simulink model "StandTurn_Balance_zhengqi"  (R2021a)
settings: Solver=FixedStepDiscrete  StartTime=0.0  StopTime=inf  FixedStep=0.0005  RelTol=1e-3
libraries: simulink x13, IFR_StackLiteDualDrive_SimulinkLib x4
settings Model: Creator=ysl  LastModifiedBy=ysl
settings OptimizationCC: DefaultParameterBehavior=Inlined  EnhancedBackFolding=on  PassReuseOutputArgsAs=Individual arguments  ZeroExternalMemoryAtStartup=off  ZeroInternalMemoryAtStartup=off  OptimizeBlockOrder=speed  DifferentSizesBufferReuse=on  OptimizationCustomize=off  EfficientTunableParamExpr=on
settings DebuggingCC: ParameterTunabilityLossMsg=error
settings SFSimCC: MATLABDynamicMemAlloc=off
settings RTWCC: Description=IFR StackLite-DualDrive Base on stm32f405RGT6  SystemTargetFile=stacklite_dualdrive.tlc  TemplateMakefile=stacklite_dualdrive.tmf  GenerateReport=on
settings CodeAppCC: ForceParamTrailComments=on  IgnoreCustomStorageClasses=off  OperatorAnnotations=on  SimulinkDataObjDesc=on  SFDataObjDesc=on  InsertBlockDesc=on
settings STFCustomTargetCC: TargetLangStandard=C99 (ISO)  MultiwordLength=256  ParMdlRefBuildCompliant=on  CompOptLevelCompliant=on  CombineOutputUpdateFcns=on  ERTCustomFileBanners=on  SupportContinuousTime=off  SupportNonInlinedSFcns=off  RemoveResetFunc=on  MATLABClassNameForMDSCustomization=Simulink.SoftwareTarget.ERTCustomization  CPPClassGenCompliant=on  GRTInterface=off  UseToolchainInfoCompliant=off  SystemTargetFile=stacklite_dualdrive.tlc
settings ERTTargetCC: TargetLangStandard=C99 (ISO)  ConcurrentExecutionCompliant=off  ModelStepFunctionPrototypeControlCompliant=off  UseToolchainInfoCompliant=off  InlinedParameterPlacement=NonHierarchical  ERTCustomFileTemplate=example_file_process.tlc

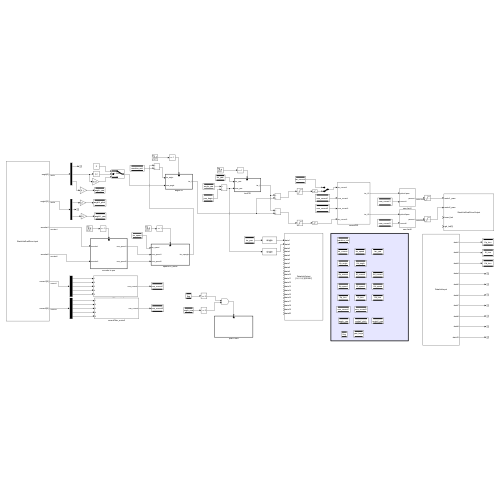
[thumbnail: Simulink's stored preview of the top-level diagram]
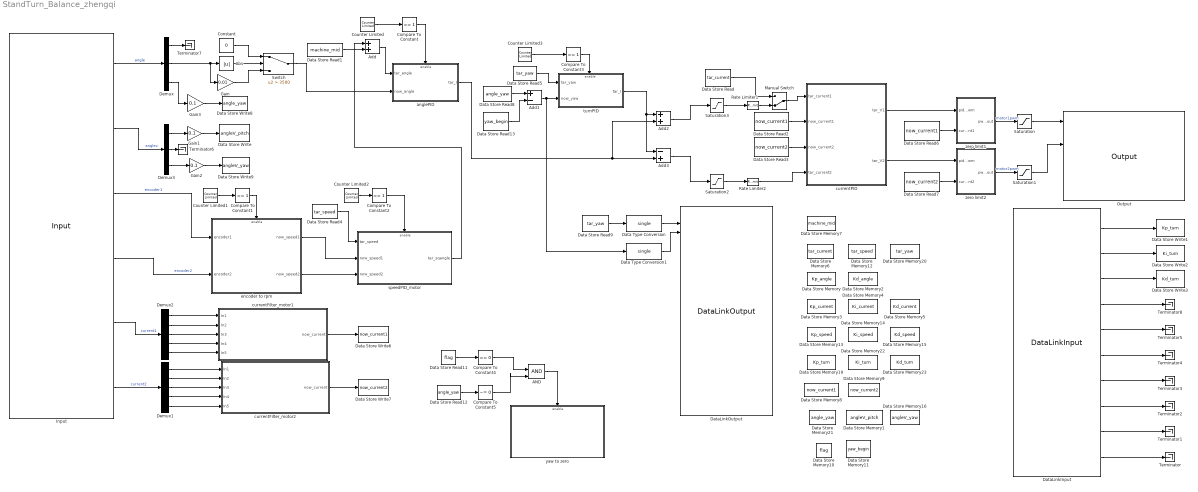
== system StandTurn_Balance_zhengqi ==
  AND : Logic  IconShape=distinctive  AllPortsSameDT=off  OutDataTypeStr=boolean
  Abs : Abs
  Add : Sum
  Add1 : Sum  Inputs=+-
  Add2 : Sum
  Add3 : Sum  Inputs=-+
  Compare To Constant{,1..3} (4 alike) : simulink/Logic and Bit Operations/Compare To Constant  relop===  const=1  OutDataTypeStr=boolean
  Compare To Constant4 : simulink/Logic and Bit Operations/Compare To Constant  relop===  const=0  OutDataTypeStr=boolean
  Compare To Constant5 : simulink/Logic and Bit Operations/Compare To Constant  relop=~=  const=0  OutDataTypeStr=boolean
  Constant : Constant  Value=0
  Counter Limited{,1..3} (4 alike) : simulink/Sources/Counter Limited  uplimit=1  tsamp=-1
  Data Store Memory : DataStoreMemory  DataStoreName=Kp_angle  ReadBeforeWriteMsg=warning  WriteAfterWriteMsg=warning  WriteAfterReadMsg=warning  ShowAdditionalParam=off
  Data Store Memory1 : DataStoreMemory  DataStoreName=angleV_pitch  ReadBeforeWriteMsg=warning  WriteAfterWriteMsg=warning  WriteAfterReadMsg=warning  ShowAdditionalParam=off
  Data Store Memory10 : DataStoreMemory  DataStoreName=flag  ReadBeforeWriteMsg=warning  WriteAfterWriteMsg=warning  WriteAfterReadMsg=warning  ShowAdditionalParam=off
  Data Store Memory11 : DataStoreMemory  DataStoreName=yaw_begin  ReadBeforeWriteMsg=warning  WriteAfterWriteMsg=warning  WriteAfterReadMsg=warning  ShowAdditionalParam=off
  Data Store Memory12 : DataStoreMemory  DataStoreName=tar_speed  ReadBeforeWriteMsg=warning  WriteAfterWriteMsg=warning  WriteAfterReadMsg=warning  ShowAdditionalParam=off
  Data Store Memory13 : DataStoreMemory  DataStoreName=Kp_speed  ReadBeforeWriteMsg=warning  WriteAfterWriteMsg=warning  WriteAfterReadMsg=warning  ShowAdditionalParam=off
  Data Store Memory14 : DataStoreMemory  DataStoreName=Ki_speed  ReadBeforeWriteMsg=warning  WriteAfterWriteMsg=warning  WriteAfterReadMsg=warning  ShowAdditionalParam=off
  Data Store Memory15 : DataStoreMemory  DataStoreName=Kd_speed  ReadBeforeWriteMsg=warning  WriteAfterWriteMsg=warning  WriteAfterReadMsg=warning  ShowAdditionalParam=off
  Data Store Memory16 : DataStoreMemory  DataStoreName=angleV_yaw  ReadBeforeWriteMsg=warning  WriteAfterWriteMsg=warning  WriteAfterReadMsg=warning  ShowAdditionalParam=off
  Data Store Memory19 : DataStoreMemory  DataStoreName=Kp_turn  ReadBeforeWriteMsg=warning  WriteAfterWriteMsg=warning  WriteAfterReadMsg=warning  ShowAdditionalParam=off
  Data Store Memory2 : DataStoreMemory  DataStoreName=Kd_angle  ReadBeforeWriteMsg=warning  WriteAfterWriteMsg=warning  WriteAfterReadMsg=warning  ShowAdditionalParam=off
  Data Store Memory20 : DataStoreMemory  DataStoreName=tar_yaw  ReadBeforeWriteMsg=warning  WriteAfterWriteMsg=warning  WriteAfterReadMsg=warning  ShowAdditionalParam=off
  Data Store Memory21 : DataStoreMemory  DataStoreName=angle_yaw  ReadBeforeWriteMsg=warning  WriteAfterWriteMsg=warning  WriteAfterReadMsg=warning  ShowAdditionalParam=off
  Data Store Memory22 : DataStoreMemory  DataStoreName=Ki_turn  ReadBeforeWriteMsg=warning  WriteAfterWriteMsg=warning  WriteAfterReadMsg=warning  ShowAdditionalParam=off
  Data Store Memory23 : DataStoreMemory  DataStoreName=Kd_turn  ReadBeforeWriteMsg=warning  WriteAfterWriteMsg=warning  WriteAfterReadMsg=warning  ShowAdditionalParam=off
  Data Store Memory3 : DataStoreMemory  DataStoreName=Kp_current  ReadBeforeWriteMsg=warning  WriteAfterWriteMsg=warning  WriteAfterReadMsg=warning  ShowAdditionalParam=off
  Data Store Memory4 : DataStoreMemory  DataStoreName=Ki_current  ReadBeforeWriteMsg=warning  WriteAfterWriteMsg=warning  WriteAfterReadMsg=warning  ShowAdditionalParam=off
  Data Store Memory5 : DataStoreMemory  DataStoreName=Kd_current  ReadBeforeWriteMsg=warning  WriteAfterWriteMsg=warning  WriteAfterReadMsg=warning  ShowAdditionalParam=off
  Data Store Memory6 : DataStoreMemory  DataStoreName=tar_current  ReadBeforeWriteMsg=warning  WriteAfterWriteMsg=warning  WriteAfterReadMsg=warning  ShowAdditionalParam=off
  Data Store Memory7 : DataStoreMemory  DataStoreName=machine_mid  ReadBeforeWriteMsg=warning  WriteAfterWriteMsg=warning  WriteAfterReadMsg=warning  ShowAdditionalParam=off
  Data Store Memory8 : DataStoreMemory  DataStoreName=now_current1  ReadBeforeWriteMsg=warning  WriteAfterWriteMsg=warning  WriteAfterReadMsg=warning  ShowAdditionalParam=off
  Data Store Memory9 : DataStoreMemory  DataStoreName=now_current2  ReadBeforeWriteMsg=warning  WriteAfterWriteMsg=warning  WriteAfterReadMsg=warning  ShowAdditionalParam=off
  Data Store Read : DataStoreRead  DataStoreName=tar_current  IndexOptions=Index vector (dialog)  Indices=1  OutputSizes=1
  Data Store Read1 : DataStoreRead  DataStoreName=machine_mid  IndexOptions=Index vector (dialog)  Indices=1  OutputSizes=1
  Data Store Read11 : DataStoreRead  DataStoreName=flag  IndexOptions=Index vector (dialog)  Indices=1  OutputSizes=1
  Data Store Read12 : DataStoreRead  DataStoreName=angle_yaw  IndexOptions=Index vector (dialog)  Indices=1  OutputSizes=1
  Data Store Read13 : DataStoreRead  DataStoreName=yaw_begin  IndexOptions=Index vector (dialog)  Indices=1  OutputSizes=1
  Data Store Read2 : DataStoreRead  DataStoreName=now_current1  IndexOptions=Index vector (dialog)  Indices=1  OutputSizes=1
  Data Store Read3 : DataStoreRead  DataStoreName=now_current2  IndexOptions=Index vector (dialog)  Indices=1  OutputSizes=1
  Data Store Read4 : DataStoreRead  DataStoreName=tar_speed  IndexOptions=Index vector (dialog)  Indices=1  OutputSizes=1
  Data Store Read5 : DataStoreRead  DataStoreName=tar_yaw  IndexOptions=Index vector (dialog)  Indices=1  OutputSizes=1
  Data Store Read6 : DataStoreRead  DataStoreName=now_current1  IndexOptions=Index vector (dialog)  Indices=1  OutputSizes=1
  Data Store Read7 : DataStoreRead  DataStoreName=now_current2  IndexOptions=Index vector (dialog)  Indices=1  OutputSizes=1
  Data Store Read8 : DataStoreRead  DataStoreName=angle_yaw  IndexOptions=Index vector (dialog)  Indices=1  OutputSizes=1
  Data Store Read9 : DataStoreRead  DataStoreName=tar_yaw  IndexOptions=Index vector (dialog)  Indices=1  OutputSizes=1
  Data Store Write : DataStoreWrite  DataStoreName=angleV_pitch  IndexOptions=Index vector (dialog)  Indices=1  OutputSizes=1
  Data Store Write1 : DataStoreWrite  DataStoreName=Kp_turn  IndexOptions=Index vector (dialog)  Indices=1  OutputSizes=1
  Data Store Write2 : DataStoreWrite  DataStoreName=Ki_turn  IndexOptions=Index vector (dialog)  Indices=1  OutputSizes=1
  Data Store Write3 : DataStoreWrite  DataStoreName=Kd_turn  IndexOptions=Index vector (dialog)  Indices=1  OutputSizes=1
  Data Store Write6 : DataStoreWrite  DataStoreName=now_current1  IndexOptions=Index vector (dialog)  Indices=1  OutputSizes=1
  Data Store Write7 : DataStoreWrite  DataStoreName=now_current2  IndexOptions=Index vector (dialog)  Indices=1  OutputSizes=1
  Data Store Write8 : DataStoreWrite  DataStoreName=angle_yaw  IndexOptions=Index vector (dialog)  Indices=1  OutputSizes=1
  Data Store Write9 : DataStoreWrite  DataStoreName=angleV_yaw  IndexOptions=Index vector (dialog)  Indices=1  OutputSizes=1
  Data Type Conversion : DataTypeConversion  OutDataTypeStr=single
  Data Type Conversion1 : DataTypeConversion  OutDataTypeStr=single
  DataLinkInput : IFR_StackLiteDualDrive_SimulinkLib/DataLinkInput
      settings: SourceProductName=IFR_StackLiteDualDrive_SimulinkLib_V1.0
  DataLinkOutput : IFR_StackLiteDualDrive_SimulinkLib/DataLinkOutput  id='BalanceUnname'  key='IFR00'
      settings: SourceProductName=IFR_StackLiteDualDrive_SimulinkLib_V1.0
  Demux : Demux  Outputs=3
  Demux1 : Demux  Outputs=5
  Demux2 : Demux  Outputs=5
  Demux3 : Demux  Outputs=3
  Gain : Gain  Gain=0.01
  Gain1 : Gain  Gain=0.1
  Gain2 : Gain  Gain=0.1
  Gain3 : Gain  Gain=0.1
  Input : IFR_StackLiteDualDrive_SimulinkLib/Input  Priority=0
      settings: SourceProductName=IFR_StackLiteDualDrive_SimulinkLib_V1.0
  Manual Switch : ManualSwitch  CurrentSetting=0
  Output : IFR_StackLiteDualDrive_SimulinkLib/Output  Priority=255
      settings: SourceProductName=IFR_StackLiteDualDrive_SimulinkLib_V1.0
  Rate Limiter1 : RateLimiter  RisingSlewLimit=10000  FallingSlewLimit=-10000  SampleTimeMode=inherited
  Rate Limiter2 : RateLimiter  RisingSlewLimit=10000  FallingSlewLimit=-10000  SampleTimeMode=inherited
  Saturation : Saturate  UpperLimit=4200  LowerLimit=-4200
  Saturation1 : Saturate  UpperLimit=4200  LowerLimit=-4200
  Saturation2 : Saturate  UpperLimit=2048  LowerLimit=-2048  OutDataTypeStr=int16
  Saturation3 : Saturate  UpperLimit=2048  LowerLimit=-2048  OutDataTypeStr=int16
  Switch : Switch  Criteria=u2 > Threshold  Threshold=3500
  Terminator{,1..8} (9 alike) : Terminator
  anglePID : Subsystem
  currentFilter_motor1 : Subsystem
  currentFilter_motor2 : Subsystem
  currentPID : Subsystem
  encoder to rpm : Subsystem
  speedPID_motor : Subsystem
  turnPID : Subsystem
  yaw to zero : Subsystem
  zero limit1 : Subsystem
  zero limit2 : Subsystem
  wires:
  Input/5 -> Demux2/1  "current1"
  Saturation1/1 -> Output/2
  Saturation2/1 -> Rate Limiter2/1
  Data Store Read3/1 -> currentPID/3(now_current2)
  Rate Limiter2/1 -> currentPID/4(tar_current2)
  Input/1 -> Demux/1  "angle"
  currentFilter_motor2/1(now_current) -> Data Store Write7/1
  Manual Switch/1 -> currentPID/1(tar_current1)
  Compare To Constant1/1 -> encoder to rpm/Enable
  Demux1/4 -> currentFilter_motor2/4(In4)
  Counter Limited1/1 -> Compare To Constant1/1
  Demux2/2 -> currentFilter_motor1/2(In2)
  zero limit2/1(pwmout) -> Saturation1/1  "motor2pwm"
  Demux1/1 -> currentFilter_motor2/1(In1)
  Demux2/5 -> currentFilter_motor1/5(In5)
  Input/3 -> encoder to rpm/1(encoder1)  "encoder1"
  Saturation3/1 -> Rate Limiter1/1
  Saturation/1 -> Output/1
  Demux1/3 -> currentFilter_motor2/3(In3)
  Input/6 -> Demux1/1  "current2"
  Demux2/3 -> currentFilter_motor1/3(In3)
  Demux/3 -> Gain3/1
  currentPID/2(tar_V2) -> zero limit2/1(pidout2pwm)
  Input/2 -> Demux3/1  "anglev"
  Demux3/2 -> Terminator6/1
  Demux2/1 -> currentFilter_motor1/1(In1)
  Demux1/5 -> currentFilter_motor2/5(In5)
  Input/4 -> encoder to rpm/2(encoder2)  "encoder2"
  currentPID/1(tar_V1) -> zero limit1/1(pidout1pwm)
  Demux1/2 -> currentFilter_motor2/2(In2)
  Data Store Read2/1 -> currentPID/2(now_current1)
  Data Store Read7/1 -> zero limit2/2(current2)
  currentFilter_motor1/1(now_current) -> Data Store Write6/1
  Rate Limiter1/1 -> Manual Switch/2
  Demux2/4 -> currentFilter_motor1/4(In4)
  zero limit1/1(pwmout) -> Saturation/1  "motor1pwm"
  Data Store Read/1 -> Manual Switch/1
  Data Store Read6/1 -> zero limit1/2(current1)
  Add/1 -> anglePID/1(tar_angle)
  Abs/1 -> Switch/2
  Gain/1 -> Switch/3
  Constant/1 -> Switch/1
  Demux/2 -> Gain/1, Abs/1
  Counter Limited/1 -> Compare To Constant/1
  Switch/1 -> anglePID/2(now_angle)
  Data Store Read1/1 -> Add/2
  Compare To Constant/1 -> anglePID/Enable
  Demux/1 -> Terminator7/1
  speedPID_motor/1(tar_sqangle) -> Add/1
  Demux3/1 -> Gain1/1
  Gain1/1 -> Data Store Write/1
  Data Store Read4/1 -> speedPID_motor/1(tar_speed)
  Counter Limited2/1 -> Compare To Constant2/1
  Compare To Constant2/1 -> speedPID_motor/Enable
  encoder to rpm/1(now_speed1) -> speedPID_motor/2(now_speed1)
  encoder to rpm/2(now_speed2) -> speedPID_motor/3(now_speed2)
  Data Store Read5/1 -> turnPID/1(tar_yaw)
  Demux3/3 -> Gain2/1
  Gain2/1 -> Data Store Write9/1
  Gain3/1 -> Data Store Write8/1
  turnPID/1(tar_I) -> Add3/1, Add2/1
  anglePID/1(tar_I) -> Add2/2, Add3/2
  Add2/1 -> Saturation3/1
  Add3/1 -> Saturation2/1
  Compare To Constant3/1 -> turnPID/Enable
  Counter Limited3/1 -> Compare To Constant3/1
  Data Store Read9/1 -> Data Type Conversion/1
  Data Type Conversion/1 -> DataLinkOutput/1
  Add1/1 -> Data Type Conversion1/1, turnPID/2(now_yaw)
  Data Type Conversion1/1 -> DataLinkOutput/2
  Data Store Read11/1 -> Compare To Constant4/1
  Data Store Read12/1 -> Compare To Constant5/1
  Compare To Constant4/1 -> AND/1
  Compare To Constant5/1 -> AND/2
  AND/1 -> yaw to zero/Enable
  Data Store Read8/1 -> Add1/1
  Data Store Read13/1 -> Add1/2
  DataLinkInput/10 -> Terminator/1
  DataLinkInput/9 -> Terminator1/1
  DataLinkInput/8 -> Terminator2/1
  DataLinkInput/7 -> Terminator3/1
  DataLinkInput/6 -> Terminator4/1
  DataLinkInput/5 -> Terminator5/1
  DataLinkInput/4 -> Terminator8/1
  DataLinkInput/1 -> Data Store Write1/1
  DataLinkInput/2 -> Data Store Write2/1
  DataLinkInput/3 -> Data Store Write3/1

== system StandTurn_Balance_zhengqi/anglePID ==
  tar_angle : Inport
  now_angle : Inport  Port=2
  Enable : EnablePort
  Add : Sum  OutDataTypeStr=double
  Add1 : Sum  Inputs=+-
  D : Subsystem
  P : Subsystem
  tar_I : Outport
  wires:
  Add/1 -> tar_I/1
  D/1(Out1) -> Add/2
  now_angle/1 -> Add1/2
  tar_angle/1 -> Add1/1
  P/1(Out1) -> Add/1
  Add1/1 -> P/1(error)

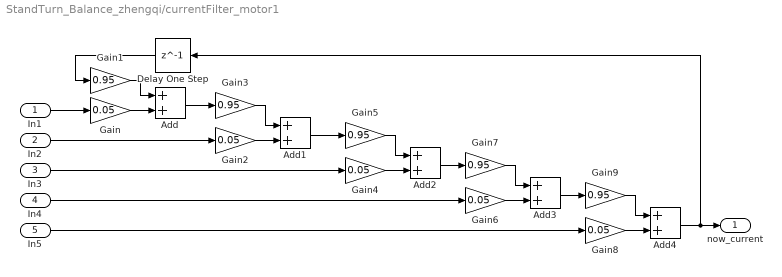
== system StandTurn_Balance_zhengqi/currentFilter_motor1 ==
  In1 : Inport
  In2 : Inport  Port=2
  In3 : Inport  Port=3
  In4 : Inport  Port=4
  In5 : Inport  Port=5
  Add{,1..4} (5 alike) : Sum
  Delay One Step : Delay  DelayLength=1
  Gain{,2,4,6,8} (5 alike) : Gain  Gain=0.05  OutDataTypeStr=single
  Gain{1,3,5,7,9} (5 alike) : Gain  Gain=0.95  OutDataTypeStr=single
  now_current : Outport
  wires:
  Gain1/1 -> Add/1
  Gain5/1 -> Add2/1
  Gain/1 -> Add/2
  Gain3/1 -> Add1/1
  In2/1 -> Gain2/1
  Gain2/1 -> Add1/2
  Delay One Step/1 -> Gain1/1
  In1/1 -> Gain/1
  Add/1 -> Gain3/1
  Gain4/1 -> Add2/2
  In4/1 -> Gain6/1
  Add1/1 -> Gain5/1
  Gain9/1 -> Add4/1
  Add2/1 -> Gain7/1
  Gain8/1 -> Add4/2
  Gain7/1 -> Add3/1
  Add4/1 -> now_current/1, Delay One Step/1
  Gain6/1 -> Add3/2
  Add3/1 -> Gain9/1
  In5/1 -> Gain8/1
  In3/1 -> Gain4/1

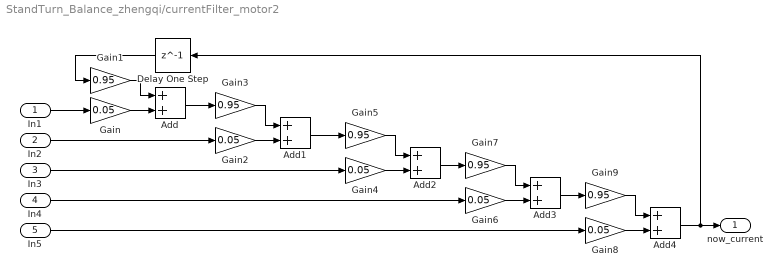
== system StandTurn_Balance_zhengqi/currentFilter_motor2 ==
  In1 : Inport
  In2 : Inport  Port=2
  In3 : Inport  Port=3
  In4 : Inport  Port=4
  In5 : Inport  Port=5
  Add{,1..4} (5 alike) : Sum
  Delay One Step : Delay  DelayLength=1
  Gain{,2,4,6,8} (5 alike) : Gain  Gain=0.05  OutDataTypeStr=single
  Gain{1,3,5,7,9} (5 alike) : Gain  Gain=0.95  OutDataTypeStr=single
  now_current : Outport
  wires:
  In3/1 -> Gain4/1
  In5/1 -> Gain8/1
  Add3/1 -> Gain9/1
  Gain6/1 -> Add3/2
  Add4/1 -> Delay One Step/1, now_current/1
  Gain7/1 -> Add3/1
  Gain8/1 -> Add4/2
  Add2/1 -> Gain7/1
  Gain9/1 -> Add4/1
  Add1/1 -> Gain5/1
  In4/1 -> Gain6/1
  Gain4/1 -> Add2/2
  Add/1 -> Gain3/1
  In1/1 -> Gain/1
  Delay One Step/1 -> Gain1/1
  Gain2/1 -> Add1/2
  In2/1 -> Gain2/1
  Gain3/1 -> Add1/1
  Gain/1 -> Add/2
  Gain5/1 -> Add2/1
  Gain1/1 -> Add/1

== system StandTurn_Balance_zhengqi/currentPID ==
  tar_current1 : Inport
  now_current1 : Inport  Port=2
  now_current2 : Inport  Port=3
  tar_current2 : Inport  Port=4
  currentPID_motor1 : Subsystem
  currentPID_motor2 : Subsystem
  tar_V1 : Outport
  tar_V2 : Outport  Port=2
  wires:
  tar_current1/1 -> currentPID_motor1/1(tar_current)
  now_current1/1 -> currentPID_motor1/2(now_current)
  currentPID_motor1/1(tar_V) -> tar_V1/1
  now_current2/1 -> currentPID_motor2/2(now_current)
  currentPID_motor2/1(tar_V) -> tar_V2/1
  tar_current2/1 -> currentPID_motor2/1(tar_current)

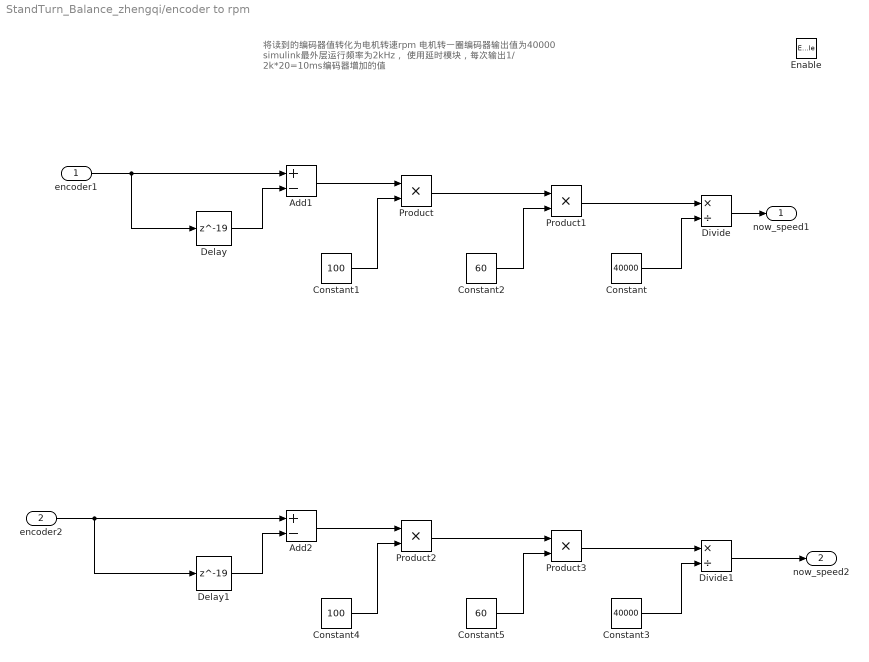
== system StandTurn_Balance_zhengqi/encoder to rpm ==
  note: 将读到的编码器值转化为电机转速rpm
      | 电机转一圈编码器输出值为40000
      | simulink最外层运行频率为2kHz，
      | 使用延时模块，每次输出1/ 2k*20=10ms编码器增加的值
  encoder1 : Inport
  encoder2 : Inport  Port=2
  Enable : EnablePort
  Add1 : Sum  Inputs=+-
  Add2 : Sum  Inputs=+-
  Constant : Constant  Value=40000  OutDataTypeStr=single
  Constant1 : Constant  Value=100  OutDataTypeStr=single
  Constant2 : Constant  Value=60  OutDataTypeStr=single
  Constant3 : Constant  Value=40000  OutDataTypeStr=single
  Constant4 : Constant  Value=100  OutDataTypeStr=single
  Constant5 : Constant  Value=60  OutDataTypeStr=single
  Delay : Delay  DelayLength=19
  Delay1 : Delay  DelayLength=19
  Divide : Product  Inputs=*/  OutDataTypeStr=single
  Divide1 : Product  Inputs=*/  OutDataTypeStr=single
  Product{,1..3} (4 alike) : Product  OutDataTypeStr=single
  now_speed1 : Outport
  now_speed2 : Outport  Port=2
  wires:
  Product1/1 -> Divide/1
  Product/1 -> Product1/1
  Constant/1 -> Divide/2
  encoder1/1 -> Add1/1, Delay/1
  Add2/1 -> Product2/1
  Delay1/1 -> Add2/2
  encoder2/1 -> Add2/1, Delay1/1
  Constant1/1 -> Product/2
  Add1/1 -> Product/1
  Constant2/1 -> Product1/2
  Delay/1 -> Add1/2
  Divide1/1 -> now_speed2/1
  Product2/1 -> Product3/1
  Constant4/1 -> Product2/2
  Product3/1 -> Divide1/1
  Constant5/1 -> Product3/2
  Divide/1 -> now_speed1/1
  Constant3/1 -> Divide1/2

== system StandTurn_Balance_zhengqi/speedPID_motor ==
  tar_speed : Inport
  now_speed1 : Inport  Port=2
  now_speed2 : Inport  Port=3
  Enable : EnablePort
  Subsystem2 : Subsystem
  tar_sqangle : Outport
  wires:
  Subsystem2/1(tar_sqangle) -> tar_sqangle/1
  now_speed2/1 -> Subsystem2/3(now_speed2)
  now_speed1/1 -> Subsystem2/2(now_speed1)
  tar_speed/1 -> Subsystem2/1(tar_speed)

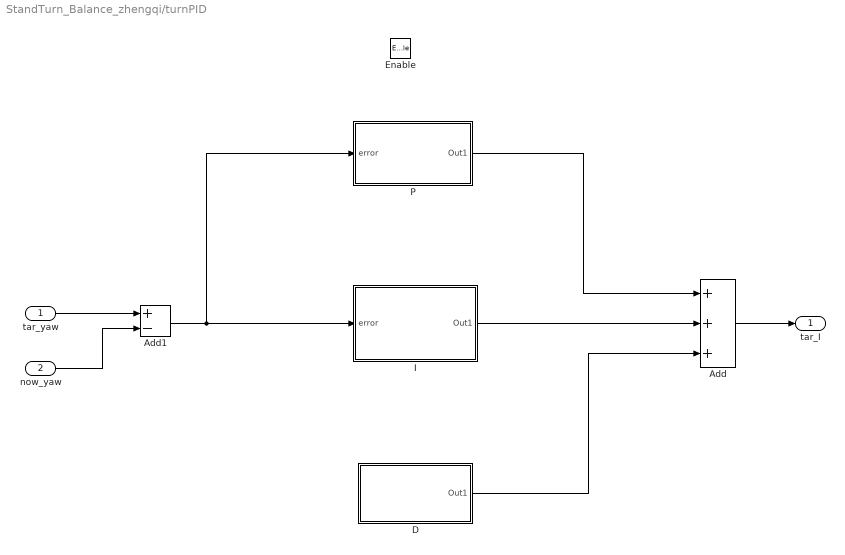
== system StandTurn_Balance_zhengqi/turnPID ==
  tar_yaw : Inport
  now_yaw : Inport  Port=2
  Enable : EnablePort
  Add : Sum  Inputs=+++  OutDataTypeStr=double
  Add1 : Sum  Inputs=+-
  D : Subsystem
  I : Subsystem
  P : Subsystem
  tar_I : Outport
  wires:
  I/1(Out1) -> Add/2
  tar_yaw/1 -> Add1/1
  now_yaw/1 -> Add1/2
  P/1(Out1) -> Add/1
  Add1/1 -> I/1(error), P/1(error)
  Add/1 -> tar_I/1
  D/1(Out1) -> Add/3

== system StandTurn_Balance_zhengqi/yaw to zero ==
  Enable : EnablePort
  Constant : Constant
  Data Store Read : DataStoreRead  DataStoreName=angle_yaw  IndexOptions=Index vector (dialog)  Indices=1  OutputSizes=1
  Data Store Write : DataStoreWrite  DataStoreName=yaw_begin  IndexOptions=Index vector (dialog)  Indices=1  OutputSizes=1
  Data Store Write1 : DataStoreWrite  DataStoreName=flag  IndexOptions=Index vector (dialog)  Indices=1  OutputSizes=1
  wires:
  Data Store Read/1 -> Data Store Write/1
  Constant/1 -> Data Store Write1/1

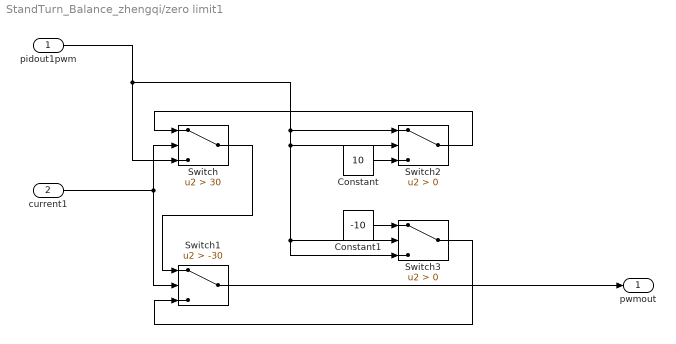
== system StandTurn_Balance_zhengqi/zero limit1 ==
  pidout1pwm : Inport
  current1 : Inport  Port=2
  Constant : Constant  Value=10  OutDataTypeStr=int16
  Constant1 : Constant  Value=-10  OutDataTypeStr=int16
  Switch : Switch  Criteria=u2 > Threshold  Threshold=30  OutDataTypeStr=int16
  Switch1 : Switch  Criteria=u2 > Threshold  Threshold=-30  OutDataTypeStr=int16
  Switch2 : Switch  Criteria=u2 > Threshold  OutDataTypeStr=int16
  Switch3 : Switch  Criteria=u2 > Threshold  OutDataTypeStr=int16
  pwmout : Outport
  wires:
  Switch1/1 -> pwmout/1
  Switch2/1 -> Switch/1
  Switch3/1 -> Switch1/3
  Switch/1 -> Switch1/1
  Constant/1 -> Switch2/3
  pidout1pwm/1 -> Switch2/2, Switch3/2, Switch3/3, Switch2/1, Switch/3
  current1/1 -> Switch1/2, Switch/2
  Constant1/1 -> Switch3/1

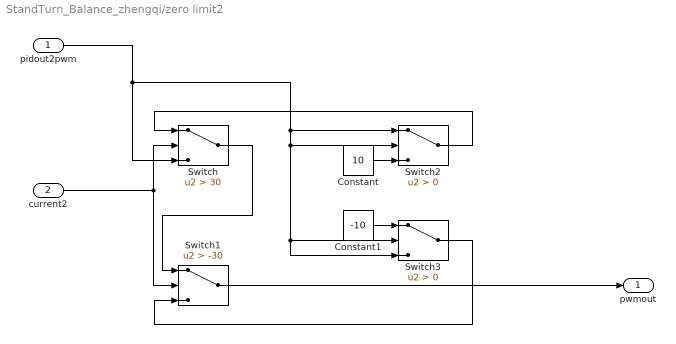
== system StandTurn_Balance_zhengqi/zero limit2 ==
  pidout2pwm : Inport
  current2 : Inport  Port=2
  Constant : Constant  Value=10  OutDataTypeStr=int16
  Constant1 : Constant  Value=-10  OutDataTypeStr=int16
  Switch : Switch  Criteria=u2 > Threshold  Threshold=30  OutDataTypeStr=int16
  Switch1 : Switch  Criteria=u2 > Threshold  Threshold=-30  OutDataTypeStr=int16
  Switch2 : Switch  Criteria=u2 > Threshold  OutDataTypeStr=int16
  Switch3 : Switch  Criteria=u2 > Threshold  OutDataTypeStr=int16
  pwmout : Outport
  wires:
  Constant1/1 -> Switch3/1
  current2/1 -> Switch/2, Switch1/2
  pidout2pwm/1 -> Switch/3, Switch2/1, Switch3/3, Switch3/2, Switch2/2
  Constant/1 -> Switch2/3
  Switch/1 -> Switch1/1
  Switch3/1 -> Switch1/3
  Switch2/1 -> Switch/1
  Switch1/1 -> pwmout/1

== system StandTurn_Balance_zhengqi/anglePID/D ==
  Constant2 : Constant  Value=0.1
  Data Store Read : DataStoreRead  DataStoreName=angleV_pitch  IndexOptions=Index vector (dialog)  Indices=1  OutputSizes=1
  Data Store Read2 : DataStoreRead  DataStoreName=Kd_angle  IndexOptions=Index vector (dialog)  Indices=1  OutputSizes=1
  Manual Switch2 : ManualSwitch
  Product2 : Product
  Out1 : Outport
  wires:
  Data Store Read/1 -> Product2/2
  Product2/1 -> Out1/1
  Data Store Read2/1 -> Manual Switch2/2
  Manual Switch2/1 -> Product2/1
  Constant2/1 -> Manual Switch2/1

== system StandTurn_Balance_zhengqi/anglePID/P ==
  error : Inport
  Constant : Constant  Value=70
  Data Store Read : DataStoreRead  DataStoreName=Kp_angle  IndexOptions=Index vector (dialog)  Indices=1  OutputSizes=1
  Manual Switch : ManualSwitch
  Product : Product
  Out1 : Outport
  wires:
  error/1 -> Product/2
  Manual Switch/1 -> Product/1
  Data Store Read/1 -> Manual Switch/2
  Constant/1 -> Manual Switch/1
  Product/1 -> Out1/1

== system StandTurn_Balance_zhengqi/currentPID/currentPID_motor1 ==
  tar_current : Inport
  now_current : Inport  Port=2
  Add : Sum  Inputs=+++  OutDataTypeStr=double
  Add1 : Sum  Inputs=+-
  D : Subsystem
  I : Subsystem
  P : Subsystem
  tar_V : Outport
  wires:
  I/1(Out1) -> Add/2
  tar_current/1 -> Add1/1
  now_current/1 -> Add1/2
  P/1(Out1) -> Add/1
  Add1/1 -> D/1(error), I/1(error), P/1(error)
  D/1(Out1) -> Add/3
  Add/1 -> tar_V/1

== system StandTurn_Balance_zhengqi/currentPID/currentPID_motor2 ==
  tar_current : Inport
  now_current : Inport  Port=2
  Add : Sum  Inputs=+++  OutDataTypeStr=double
  Add1 : Sum  Inputs=+-
  D : Subsystem
  I : Subsystem
  P : Subsystem
  tar_V : Outport
  wires:
  Add/1 -> tar_V/1
  D/1(Out1) -> Add/3
  Add1/1 -> P/1(error), I/1(error), D/1(error)
  P/1(Out1) -> Add/1
  now_current/1 -> Add1/2
  tar_current/1 -> Add1/1
  I/1(Out1) -> Add/2

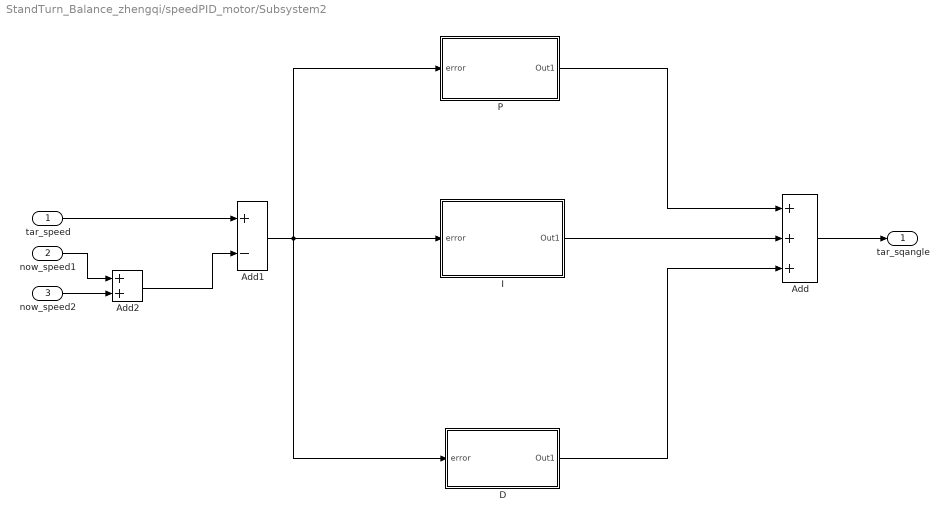
== system StandTurn_Balance_zhengqi/speedPID_motor/Subsystem2 ==
  tar_speed : Inport
  now_speed1 : Inport  Port=2
  now_speed2 : Inport  Port=3
  Add : Sum  Inputs=+++  OutDataTypeStr=double
  Add1 : Sum  Inputs=+-
  Add2 : Sum
  D : Subsystem
  I : Subsystem
  P : Subsystem
  tar_sqangle : Outport
  wires:
  Add2/1 -> Add1/2
  now_speed2/1 -> Add2/2
  now_speed1/1 -> Add2/1
  I/1(Out1) -> Add/2
  Add1/1 -> I/1(error), D/1(error), P/1(error)
  P/1(Out1) -> Add/1
  D/1(Out1) -> Add/3
  Add/1 -> tar_sqangle/1
  tar_speed/1 -> Add1/1

== system StandTurn_Balance_zhengqi/turnPID/D ==
  Constant2 : Constant  Value=0.1
  Data Store Read : DataStoreRead  DataStoreName=angleV_yaw  IndexOptions=Index vector (dialog)  Indices=1  OutputSizes=1
  Data Store Read2 : DataStoreRead  DataStoreName=Kd_turn  IndexOptions=Index vector (dialog)  Indices=1  OutputSizes=1
  Manual Switch2 : ManualSwitch  CurrentSetting=0
  Product2 : Product
  Out1 : Outport
  wires:
  Data Store Read/1 -> Product2/2
  Product2/1 -> Out1/1
  Data Store Read2/1 -> Manual Switch2/2
  Manual Switch2/1 -> Product2/1
  Constant2/1 -> Manual Switch2/1

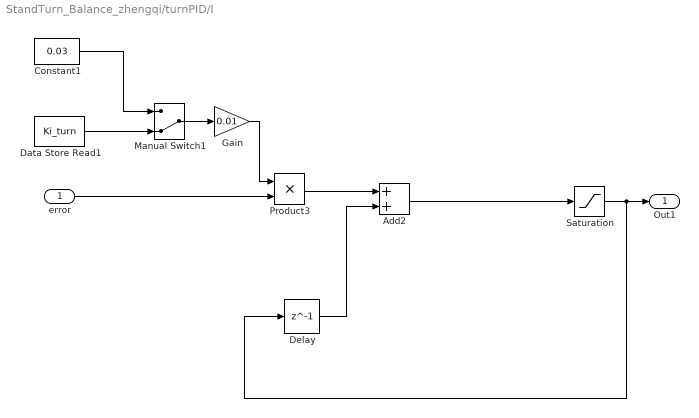
== system StandTurn_Balance_zhengqi/turnPID/I ==
  error : Inport
  Add2 : Sum
  Constant1 : Constant  Value=0.03
  Data Store Read1 : DataStoreRead  DataStoreName=Ki_turn  IndexOptions=Index vector (dialog)  Indices=1  OutputSizes=1
  Delay : Delay  DelayLength=1
  Gain : Gain  Gain=0.01
  Manual Switch1 : ManualSwitch  CurrentSetting=0
  Product3 : Product  OutDataTypeStr=single
  Saturation : Saturate  UpperLimit=2000  LowerLimit=-2000
  Out1 : Outport
  wires:
  Delay/1 -> Add2/2
  Gain/1 -> Product3/1
  Constant1/1 -> Manual Switch1/1
  Manual Switch1/1 -> Gain/1
  Data Store Read1/1 -> Manual Switch1/2
  Product3/1 -> Add2/1
  error/1 -> Product3/2
  Add2/1 -> Saturation/1
  Saturation/1 -> Delay/1, Out1/1

== system StandTurn_Balance_zhengqi/turnPID/P ==
  error : Inport
  Constant : Constant  Value=-30
  Data Store Read : DataStoreRead  DataStoreName=Kp_turn  IndexOptions=Index vector (dialog)  Indices=1  OutputSizes=1
  Manual Switch : ManualSwitch  CurrentSetting=0
  Product : Product
  Out1 : Outport
  wires:
  error/1 -> Product/2
  Manual Switch/1 -> Product/1
  Data Store Read/1 -> Manual Switch/2
  Constant/1 -> Manual Switch/1
  Product/1 -> Out1/1

== system StandTurn_Balance_zhengqi/currentPID/currentPID_motor1/D ==
  error : Inport
  Constant2 : Constant  Value=5
  Data Store Read2 : DataStoreRead  DataStoreName=Kd_current  IndexOptions=Index vector (dialog)  Indices=1  OutputSizes=1
  Difference : simulink/Discrete/Difference  ICPrevInput=0.0  OutMin=[]  OutMax=[]  OutDataType=fixdt(1, 16)  OutScaling=2^-10  DoSatur=off
  Manual Switch2 : ManualSwitch
  Product2 : Product
  Out1 : Outport
  wires:
  Difference/1 -> Product2/2
  Product2/1 -> Out1/1
  Data Store Read2/1 -> Manual Switch2/2
  Manual Switch2/1 -> Product2/1
  Constant2/1 -> Manual Switch2/1
  error/1 -> Difference/1

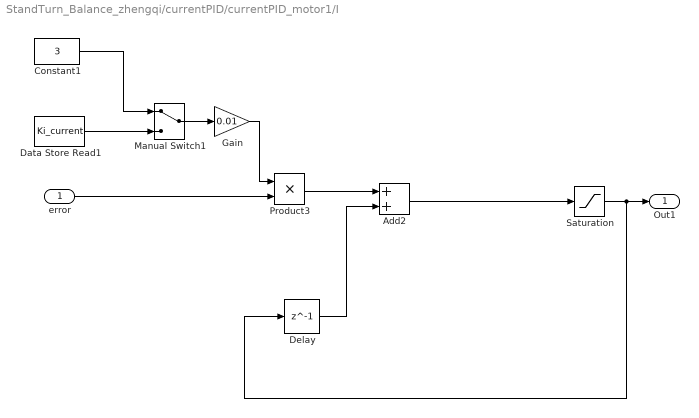
== system StandTurn_Balance_zhengqi/currentPID/currentPID_motor1/I ==
  error : Inport
  Add2 : Sum
  Constant1 : Constant  Value=3
  Data Store Read1 : DataStoreRead  DataStoreName=Ki_current  IndexOptions=Index vector (dialog)  Indices=1  OutputSizes=1
  Delay : Delay  DelayLength=1
  Gain : Gain  Gain=0.01
  Manual Switch1 : ManualSwitch
  Product3 : Product  OutDataTypeStr=single
  Saturation : Saturate  UpperLimit=2000  LowerLimit=-2000
  Out1 : Outport
  wires:
  Delay/1 -> Add2/2
  Gain/1 -> Product3/1
  Constant1/1 -> Manual Switch1/1
  Manual Switch1/1 -> Gain/1
  Data Store Read1/1 -> Manual Switch1/2
  Product3/1 -> Add2/1
  error/1 -> Product3/2
  Add2/1 -> Saturation/1
  Saturation/1 -> Delay/1, Out1/1

== system StandTurn_Balance_zhengqi/currentPID/currentPID_motor1/P ==
  error : Inport
  Constant : Constant  Value=7
  Data Store Read : DataStoreRead  DataStoreName=Kp_current  IndexOptions=Index vector (dialog)  Indices=1  OutputSizes=1
  Manual Switch : ManualSwitch
  Product : Product
  Out1 : Outport
  wires:
  error/1 -> Product/2
  Manual Switch/1 -> Product/1
  Data Store Read/1 -> Manual Switch/2
  Constant/1 -> Manual Switch/1
  Product/1 -> Out1/1

== system StandTurn_Balance_zhengqi/currentPID/currentPID_motor2/D ==
  error : Inport
  Constant2 : Constant  Value=4
  Data Store Read2 : DataStoreRead  DataStoreName=Kd_current  IndexOptions=Index vector (dialog)  Indices=1  OutputSizes=1
  Difference : simulink/Discrete/Difference  ICPrevInput=0.0  OutMin=[]  OutMax=[]  OutDataType=fixdt(1, 16)  OutScaling=2^-10  DoSatur=off
  Manual Switch2 : ManualSwitch
  Product2 : Product
  Out1 : Outport
  wires:
  error/1 -> Difference/1
  Constant2/1 -> Manual Switch2/1
  Manual Switch2/1 -> Product2/1
  Data Store Read2/1 -> Manual Switch2/2
  Product2/1 -> Out1/1
  Difference/1 -> Product2/2

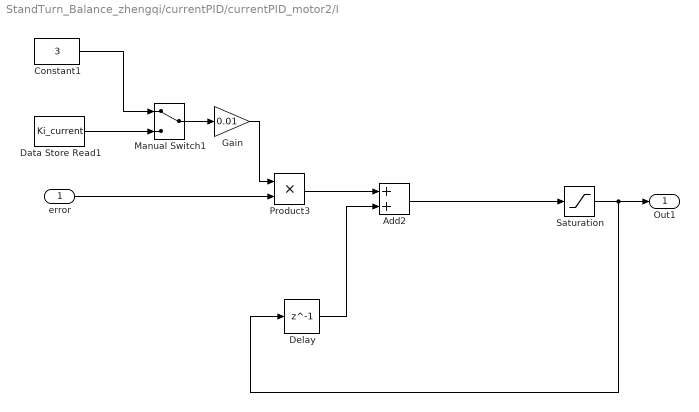
== system StandTurn_Balance_zhengqi/currentPID/currentPID_motor2/I ==
  error : Inport
  Add2 : Sum
  Constant1 : Constant  Value=3
  Data Store Read1 : DataStoreRead  DataStoreName=Ki_current  IndexOptions=Index vector (dialog)  Indices=1  OutputSizes=1
  Delay : Delay  DelayLength=1
  Gain : Gain  Gain=0.01
  Manual Switch1 : ManualSwitch
  Product3 : Product  OutDataTypeStr=single
  Saturation : Saturate  UpperLimit=2000  LowerLimit=-2000
  Out1 : Outport
  wires:
  Add2/1 -> Saturation/1
  error/1 -> Product3/2
  Product3/1 -> Add2/1
  Data Store Read1/1 -> Manual Switch1/2
  Manual Switch1/1 -> Gain/1
  Constant1/1 -> Manual Switch1/1
  Gain/1 -> Product3/1
  Delay/1 -> Add2/2
  Saturation/1 -> Out1/1, Delay/1

== system StandTurn_Balance_zhengqi/currentPID/currentPID_motor2/P ==
  error : Inport
  Constant : Constant  Value=7
  Data Store Read : DataStoreRead  DataStoreName=Kp_current  IndexOptions=Index vector (dialog)  Indices=1  OutputSizes=1
  Manual Switch : ManualSwitch
  Product : Product
  Out1 : Outport
  wires:
  Product/1 -> Out1/1
  Constant/1 -> Manual Switch/1
  Data Store Read/1 -> Manual Switch/2
  Manual Switch/1 -> Product/1
  error/1 -> Product/2

== system StandTurn_Balance_zhengqi/speedPID_motor/Subsystem2/D ==
  error : Inport
  Constant2 : Constant  Value=-100
  Data Store Read2 : DataStoreRead  DataStoreName=Kd_speed  IndexOptions=Index vector (dialog)  Indices=1  OutputSizes=1
  Difference : simulink/Discrete/Difference  ICPrevInput=0.0  OutMin=[]  OutMax=[]  OutDataType=fixdt(1, 16)  OutScaling=2^-10  DoSatur=off
  Gain : Gain  Gain=0.001
  Manual Switch2 : ManualSwitch  CurrentSetting=0
  Product2 : Product
  Out1 : Outport
  wires:
  Difference/1 -> Product2/2
  Product2/1 -> Out1/1
  Data Store Read2/1 -> Manual Switch2/2
  Manual Switch2/1 -> Gain/1
  Constant2/1 -> Manual Switch2/1
  error/1 -> Difference/1
  Gain/1 -> Product2/1

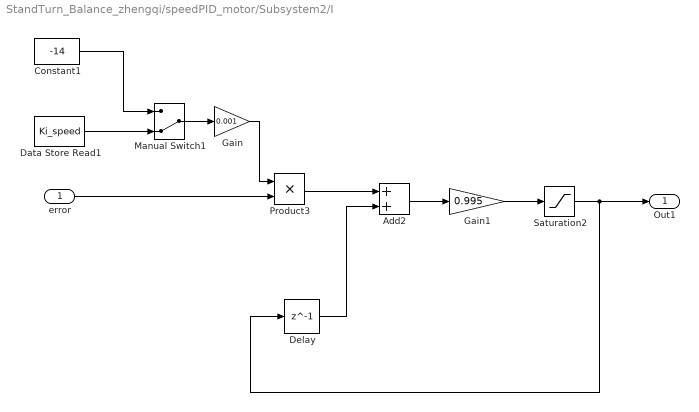
== system StandTurn_Balance_zhengqi/speedPID_motor/Subsystem2/I ==
  error : Inport
  Add2 : Sum
  Constant1 : Constant  Value=-14
  Data Store Read1 : DataStoreRead  DataStoreName=Ki_speed  IndexOptions=Index vector (dialog)  Indices=1  OutputSizes=1
  Delay : Delay  DelayLength=1
  Gain : Gain  Gain=0.001
  Gain1 : Gain  Gain=0.995
  Manual Switch1 : ManualSwitch  CurrentSetting=0
  Product3 : Product  OutDataTypeStr=single
  Saturation2 : Saturate  UpperLimit=1500  LowerLimit=-1500
  Out1 : Outport
  wires:
  Delay/1 -> Add2/2
  Gain/1 -> Product3/1
  Add2/1 -> Gain1/1
  Constant1/1 -> Manual Switch1/1
  Manual Switch1/1 -> Gain/1
  Data Store Read1/1 -> Manual Switch1/2
  Gain1/1 -> Saturation2/1
  Product3/1 -> Add2/1
  error/1 -> Product3/2
  Saturation2/1 -> Out1/1, Delay/1

== system StandTurn_Balance_zhengqi/speedPID_motor/Subsystem2/P ==
  error : Inport
  Constant : Constant  Value=-4
  Data Store Read : DataStoreRead  DataStoreName=Kp_speed  IndexOptions=Index vector (dialog)  Indices=1  OutputSizes=1
  Gain : Gain  Gain=0.001
  Manual Switch : ManualSwitch  CurrentSetting=0
  Product : Product
  Out1 : Outport
  wires:
  error/1 -> Product/2
  Data Store Read/1 -> Manual Switch/2
  Constant/1 -> Manual Switch/1
  Product/1 -> Out1/1
  Manual Switch/1 -> Gain/1
  Gain/1 -> Product/1
